simulink model "HESS"  (R2023a)
settings: Solver=daessc  StartTime=0.0  StopTime=2474  MaxStep=0.1  RelTol=1e-3
undefined symbols (not defined in the file or in its folder): Battery, Capacitor, Ri
libraries: fl_lib x31, nesl_utility x18, batteryecm_lib x1, rllib x1
settings Model: Creator=antaeug  LastModifiedBy=antaeug

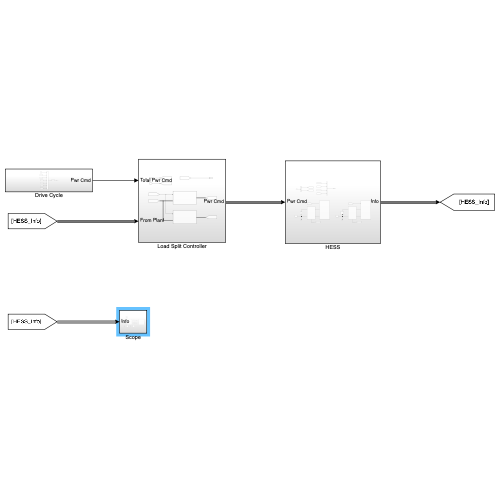
[thumbnail: Simulink's stored preview of the top-level diagram]
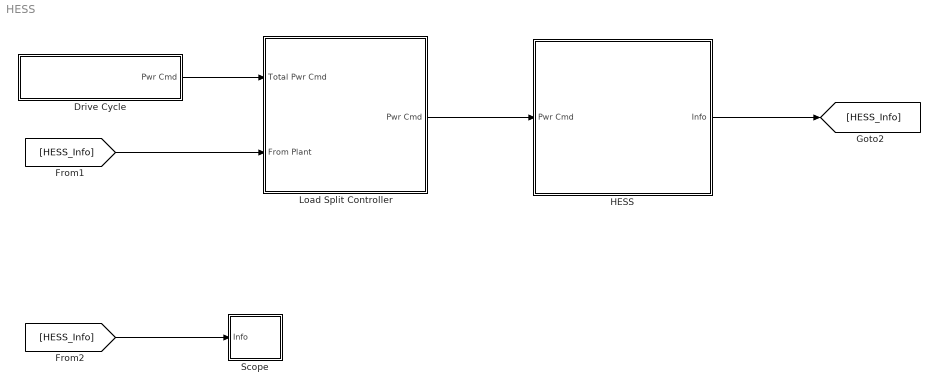
== system HESS ==
  Drive Cycle : Subsystem
  HESS : Subsystem
  Load Split Controller : Subsystem
  Scope : Subsystem
  wires:
  Drive Cycle/1(Pwr Cmd) -> Load Split Controller/1(Total Pwr Cmd)
  Load Split Controller/1(Pwr Cmd) -> HESS/1(Pwr Cmd)
  HESS/1(Info) -> [HESS_Info]
  [HESS_Info] -> Scope/1(Info)
  [HESS_Info] -> Load Split Controller/2(From Plant)

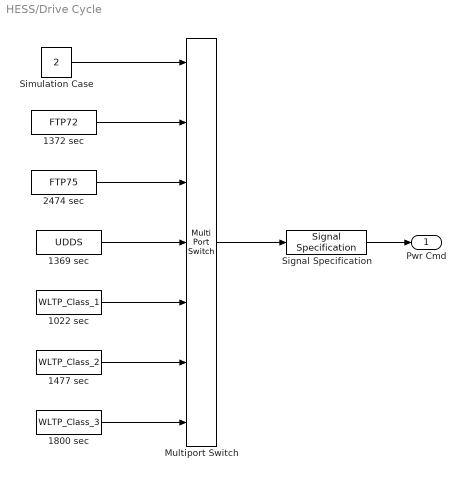
== system HESS/Drive Cycle ==
  1022 sec : FromWorkspace  VariableName=WLTP_Class_1  Interpolate=off  ZeroCross=off  OutputAfterFinalValue=Setting to zero
  1369 sec : FromWorkspace  VariableName=UDDS  Interpolate=off  ZeroCross=off  OutputAfterFinalValue=Setting to zero
  1372 sec : FromWorkspace  VariableName=FTP72  Interpolate=off  ZeroCross=off  OutputAfterFinalValue=Setting to zero
  1477 sec : FromWorkspace  VariableName=WLTP_Class_2  Interpolate=off  ZeroCross=off  OutputAfterFinalValue=Setting to zero
  1800 sec : FromWorkspace  VariableName=WLTP_Class_3  Interpolate=off  ZeroCross=off  OutputAfterFinalValue=Setting to zero
  2474 sec : FromWorkspace  VariableName=FTP75  Interpolate=off  ZeroCross=off  OutputAfterFinalValue=Setting to zero
  Multiport Switch : MultiPortSwitch  Inputs=6  SaturateOnIntegerOverflow=off  InputSameDT=off
  Signal Specification : SignalSpecification  Unit=W
  Simulation Case : Constant  Value=2
  Pwr Cmd : Outport
  wires:
  1372 sec/1 -> Multiport Switch/2
  Signal Specification/1 -> Pwr Cmd/1
  Multiport Switch/1 -> Signal Specification/1
  Simulation Case/1 -> Multiport Switch/1
  2474 sec/1 -> Multiport Switch/3
  1369 sec/1 -> Multiport Switch/4
  1477 sec/1 -> Multiport Switch/6
  1022 sec/1 -> Multiport Switch/5
  1800 sec/1 -> Multiport Switch/7

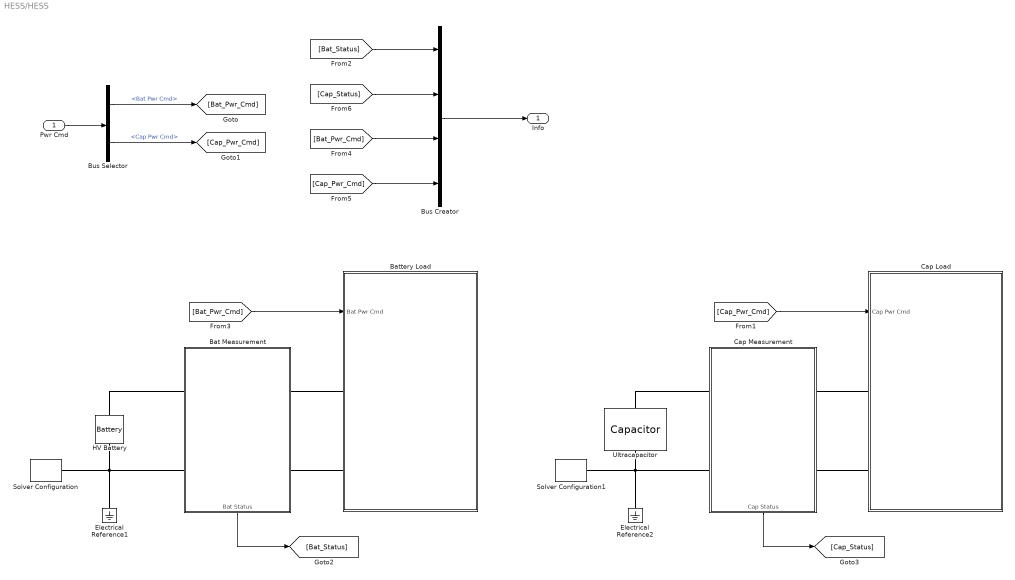
== system HESS/HESS ==
  Pwr Cmd : Inport
  Bat Measurement : Subsystem
      settings: PortSchema="{\"entries\":[{\"content\":{\"sides\":[{\"content\":{\"connectorIds\":[\"LConn1\",\"LConn2\"]},\"type\":\"ConnectorPlacement.EquallySpacedRectSide\",\"uuid\":\"d922d1f1-019d-451f-8be4-16b01e818775\"},{\"content\":{\"connectorIds\":[\"RConn1\",\"RConn2\"],\"side\":\"RIGHT\"},\"type\":\"ConnectorPlacement.EquallySpacedRectSide\",\"uuid\":\"6462d40f-4676-4bff-8e25-5b847feb4e24\"},{\"content\":{\"side\":\"TOP\"},\"type\":\"ConnectorPlacement.EquallySpacedRectSide\",\"uuid\":\"03ad4d94-013a-4b50-b094-3d1359848380\"},{\"content\":{\"connectorIds\":[\"Out1\"],\"side\":\"BOTTOM\"},\"type\":\"ConnectorPlacement.EquallySpacedRectSide\",\"uuid\":\"1e4082bc-bf86-4ee6-a4f5-78f09401198d\"}]},\"type\":\"ConnectorPlacement.EquallySpacedConnector\",\"uuid\":\"2964760f-0df3-43f8-9aa6-d9b794f3ad37\"}],\"packageUris\":[\"http://schema.mathworks.com/mf0/Connector/R2020b\"],\"version\":\"1.0\"}"
  Battery Load : Subsystem
  Bus Creator : BusCreator  Inputs=4
  Bus Selector : BusSelector  OutputSignals=Bat Pwr Cmd,Cap Pwr Cmd
  Cap Load : Subsystem
  Cap Measurement : Subsystem
      settings: PortSchema="{\"entries\":[{\"content\":{\"sides\":[{\"content\":{\"connectorIds\":[\"LConn1\",\"LConn2\"]},\"type\":\"ConnectorPlacement.EquallySpacedRectSide\",\"uuid\":\"d922d1f1-019d-451f-8be4-16b01e818775\"},{\"content\":{\"connectorIds\":[\"RConn1\",\"RConn2\"],\"side\":\"RIGHT\"},\"type\":\"ConnectorPlacement.EquallySpacedRectSide\",\"uuid\":\"6462d40f-4676-4bff-8e25-5b847feb4e24\"},{\"content\":{\"side\":\"TOP\"},\"type\":\"ConnectorPlacement.EquallySpacedRectSide\",\"uuid\":\"03ad4d94-013a-4b50-b094-3d1359848380\"},{\"content\":{\"connectorIds\":[\"Out1\"],\"side\":\"BOTTOM\"},\"type\":\"ConnectorPlacement.EquallySpacedRectSide\",\"uuid\":\"1e4082bc-bf86-4ee6-a4f5-78f09401198d\"}]},\"type\":\"ConnectorPlacement.EquallySpacedConnector\",\"uuid\":\"2964760f-0df3-43f8-9aa6-d9b794f3ad37\"}],\"packageUris\":[\"http://schema.mathworks.com/mf0/Connector/R2020b\"],\"version\":\"1.0\"}"
  Electrical Reference1 : fl_lib/Electrical/Electrical Elements/Electrical Reference
  Electrical Reference2 : fl_lib/Electrical/Electrical Elements/Electrical Reference
  HV Battery : batteryecm_lib/Battery  Vnom=Battery.NominalVoltage V  prm_dir=1  R1_dis=2 Ohm  R1_ch=2 Ohm  R1=Battery.InternalResistance Ohm  prm_AH=2  AH=Battery.Capacity hr*A  V1=Battery.V1 V  AH1=Battery.AH1 hr*A  prm_R2=1  R2=2000 Ohm  Tmeas=25 degC  charge_measurement_port=simscape.enum.battery.enable.no  prm_dyn=1  Rp1=0.005 Ohm  tau1=30 s  Rp2=0.005 Ohm  tau2=30 s  Rp3=0.005 Ohm  tau3=30 s  Rp4=0.005 Ohm  tau4=30 s  Rp5=0.005 Ohm  tau5=30 s  prm_fade=1  N_fade=100  AH_fade=45 hr*A  R1_fade=2.02 Ohm  R1_ch_fade=2.02 Ohm  V1_fade=10.35 V  prm_age=1  prm_age_OCV=1  OCV_age=0.9  SOC_age=60  Tmeas_age=298.15 K  delta_time_age_vec=[0] d  temperature_age_vec=[273] K  OCV_scaling_age=2.2134e6  OCV_offset_age=1.632e6  temp_exp_age=0.515833569 V  t_exp_age=0.75  Vnom_T2=Vnom V  R1_T2=Ri+0.1*Ri Ohm  R1_T2_dis=2.2 Ohm  R1_T2_ch=2.2 Ohm  V1_T2=V1 V  R2_T2=2200 Ohm  Rp1_T2=0.005 Ohm  tau1_T2=30 s  Rp2_T2=0.005 Ohm  tau2_T2=30 s  Rp3_T2=0.005 Ohm  tau3_T2=30 s  Rp4_T2=0.005 Ohm  tau4_T2=30 s  Rp5_T2=0.005 Ohm  tau5_T2=30 s  Tmeas2=0 degC  thermal_port=simscape.enum.thermaleffects.omit  thermal_mass=89400 J/K  i_specify=off  i_priority=None  i=0 A  i_nominal_specify=off  i_nominal_unit=A  i_nominal_value=1  v_specify=off  v_priority=None  v=0 V  v_nominal_specify=off  v_nominal_unit=V  v_nominal_value=1  charge_specify=on  charge_priority=High  charge=Battery.InitialCharge hr*A  charge_nominal_specify=off  charge_nominal_unit=A*hr  charge_nominal_value=1  num_cycles_specify=off  num_cycles_priority=High  num_cycles=0  num_cycles_nominal_specify=off  num_cycles_nominal_unit=1  num_cycles_nominal_value=1  temperature_specify=on  temperature_priority=High  temperature=25 degC  temperature_nominal_specify=off  temperature_nominal_unit=K  temperature_nominal_value=1
  Solver Configuration : nesl_utility/Solver Configuration  PhysicalDomain=network_engine_domain  SubClassName=solver  LeftPortType=input  RightPortType=generic  Tones=[]  Harmonics=[]  SimulateNoise=off  Profile=off  UseLocalSampling=off  EnableSwitchedLinearOptims=on  FrequencyDomain=off  UseCCode=off  RelTol=0.001  AbsTol=1e-06  MinStep=1e-09  ToWorkspace=off  RevertToSquareIcSolve=off  NumHomotopyIterations=100  PhasorMode=off  PhasorModeNumHarmonics=1  ConsistencySolver=NEWTON_FTOL  IndexReductionMethod=DerivativeReplacement  DoDC=off  ResidualTolerance=1e-09  ConsistencyTolSource=GLOBAL  ConsistencyAbsTol=0.001  ConsistencyRelTol=0.001  ConsistencyTolFactor=0.001  UseLocalSolver=on  LocalSolverChoice=NE_BACKWARD_EULER_ADVANCER  ResolveIndetEquations=on  FunctionEvalNumThread=1  LocalSolverSampleTime=0.01  DoFixedCost=on  MaxNonlinIter=3  MaxModeIter=2  ComputeImpulses=off  ImpulseIterations=2  LinearAlgebra=auto  LinearAlgebraNumThread=0  EquationFormulation=NE_TIME_EF  DelaysMemoryBudget=1024  AutomaticFiltering=on  FilteringTimeConstant=0.001  PartitionStorageMethod=AS_NEEDED  PartitionMemoryBudget=1024  PartitionMethod=FAST
  Solver Configuration1 : nesl_utility/Solver Configuration  PhysicalDomain=network_engine_domain  SubClassName=solver  LeftPortType=input  RightPortType=generic  Tones=[]  Harmonics=[]  SimulateNoise=off  Profile=off  UseLocalSampling=off  EnableSwitchedLinearOptims=on  FrequencyDomain=off  UseCCode=off  RelTol=0.001  AbsTol=1e-06  MinStep=1e-09  ToWorkspace=off  RevertToSquareIcSolve=off  NumHomotopyIterations=100  PhasorMode=off  PhasorModeNumHarmonics=1  ConsistencySolver=NEWTON_FTOL  IndexReductionMethod=DerivativeReplacement  DoDC=off  ResidualTolerance=1e-09  ConsistencyTolSource=GLOBAL  ConsistencyAbsTol=0.001  ConsistencyRelTol=0.001  ConsistencyTolFactor=0.001  UseLocalSolver=on  LocalSolverChoice=NE_BACKWARD_EULER_ADVANCER  ResolveIndetEquations=on  FunctionEvalNumThread=1  LocalSolverSampleTime=0.01  DoFixedCost=on  MaxNonlinIter=3  MaxModeIter=2  ComputeImpulses=off  ImpulseIterations=2  LinearAlgebra=auto  LinearAlgebraNumThread=0  EquationFormulation=NE_TIME_EF  DelaysMemoryBudget=1024  AutomaticFiltering=on  FilteringTimeConstant=0.001  PartitionStorageMethod=AS_NEEDED  PartitionMemoryBudget=1024  PartitionMethod=FAST
  Ultracapacitor : fl_lib/Electrical/Electrical Elements/Capacitor  c=Capacitor.Capacitance F  r=Capacitor.InternalResistance mOhm  g=0 1/Ohm  i_specify=off  i_priority=None  i=20 A  i_nominal_specify=off  i_nominal_unit=A  i_nominal_value=1  v_specify=off  v_priority=None  v=600 V  v_nominal_specify=off  v_nominal_unit=V  v_nominal_value=1  vc_specify=on  vc_priority=None  vc=Capacitor.Voltage V  vc_nominal_specify=off  vc_nominal_unit=V  vc_nominal_value=600
  Info : Outport
  wires:
  Pwr Cmd/1 -> Bus Selector/1
  Bus Selector/1 -> [Bat_Pwr_Cmd]  "<Bat Pwr Cmd>"
  Bus Selector/2 -> [Cap_Pwr_Cmd]  "<Cap Pwr Cmd>"
  [Bat_Status] -> Bus Creator/1
  Bus Creator/1 -> Info/1
  [Cap_Pwr_Cmd] -> Bus Creator/4
  [Bat_Pwr_Cmd] -> Bus Creator/3
  Bat Measurement/1(Bat Status) -> [Bat_Status]
  [Bat_Pwr_Cmd] -> Battery Load/1(Bat Pwr Cmd)
  Cap Measurement/1(Cap Status) -> [Cap_Status]
  [Cap_Pwr_Cmd] -> Cap Load/1(Cap Pwr Cmd)
  [Cap_Status] -> Bus Creator/2
  connections:
  HV Battery/RConn1 -- Bat Measurement/LConn2 -- Solver Configuration/RConn1 -- Electrical Reference1/LConn1
  Bat Measurement/LConn1 -- HV Battery/LConn1
  Battery Load/LConn1 -- Bat Measurement/RConn1
  Battery Load/LConn2 -- Bat Measurement/RConn2
  Electrical Reference2/LConn1 -- Ultracapacitor/RConn1 -- Cap Measurement/LConn2 -- Solver Configuration1/RConn1
  Ultracapacitor/LConn1 -- Cap Measurement/LConn1
  Cap Load/LConn2 -- Cap Measurement/RConn2
  Cap Load/LConn1 -- Cap Measurement/RConn1

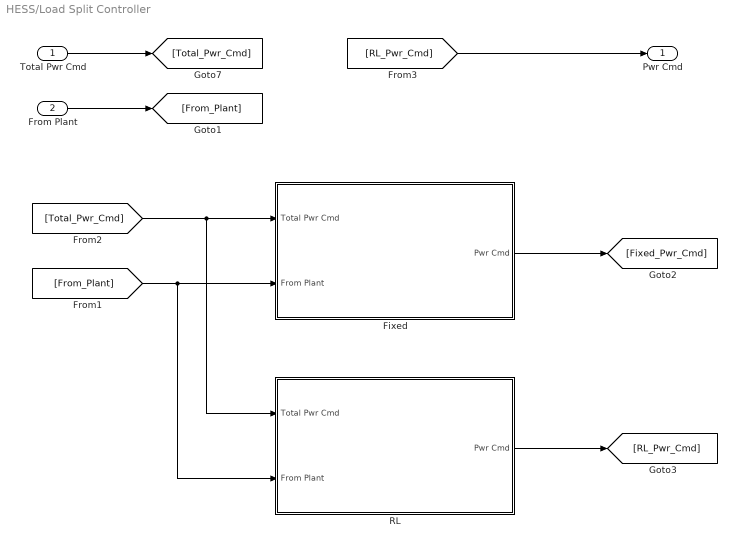
== system HESS/Load Split Controller ==
  Total Pwr Cmd : Inport
  From Plant : Inport  Port=2
  Fixed : Subsystem
  RL : Subsystem
  Pwr Cmd : Outport
  wires:
  [Total_Pwr_Cmd] -> RL/1(Total Pwr Cmd), Fixed/1(Total Pwr Cmd)
  [From_Plant] -> RL/2(From Plant), Fixed/2(From Plant)
  Fixed/1(Pwr Cmd) -> [Fixed_Pwr_Cmd]
  RL/1(Pwr Cmd) -> [RL_Pwr_Cmd]
  Total Pwr Cmd/1 -> [Total_Pwr_Cmd]
  From Plant/1 -> [From_Plant]
  [RL_Pwr_Cmd] -> Pwr Cmd/1

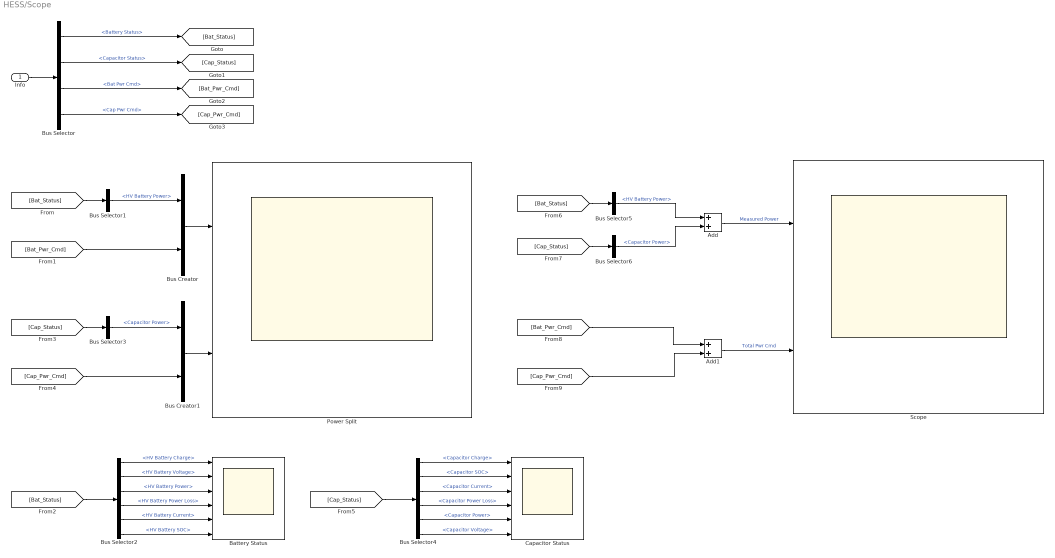
== system HESS/Scope ==
  Info : Inport
  Add : Sum
  Add1 : Sum
  Battery Status : Scope  NumInputPorts=6
  Bus Creator : BusCreator  Inputs=2
  Bus Creator1 : BusCreator  Inputs=2
  Bus Selector : BusSelector  OutputSignals=Battery Status,Capacitor Status,Bat Pwr Cmd,Cap Pwr Cmd
  Bus Selector1 : BusSelector  OutputSignals=HV Battery Power
  Bus Selector2 : BusSelector  OutputSignals=HV Battery Charge,HV Battery Voltage,HV Battery Power,HV Battery Power Loss,HV Battery Current,HV Battery SOC
  Bus Selector3 : BusSelector  OutputSignals=Capacitor Power
  Bus Selector4 : BusSelector  OutputSignals=Capacitor Charge,Capacitor SOC,Capacitor Current,Capacitor Power Loss,Capacitor Power,Capacitor Voltage
  Bus Selector5 : BusSelector  OutputSignals=HV Battery Power
  Bus Selector6 : BusSelector  OutputSignals=Capacitor Power
  Capacitor Status : Scope  NumInputPorts=6
  Power Split : Scope  NumInputPorts=2
  Scope : Scope  NumInputPorts=2
  wires:
  Info/1 -> Bus Selector/1
  Bus Selector/1 -> [Bat_Status]  "<Battery Status>"
  [Bat_Status] -> Bus Selector1/1
  Bus Selector1/1 -> Bus Creator/1  "<HV Battery Power>"
  [Bat_Pwr_Cmd] -> Bus Creator/2
  Bus Selector/3 -> [Bat_Pwr_Cmd]  "<Bat Pwr Cmd>"
  Bus Selector/4 -> [Cap_Pwr_Cmd]  "<Cap Pwr Cmd>"
  [Bat_Status] -> Bus Selector2/1
  Bus Selector2/1 -> Battery Status/1  "<HV Battery Charge>"
  Bus Selector2/2 -> Battery Status/2  "<HV Battery Voltage>"
  Bus Selector2/3 -> Battery Status/3  "<HV Battery Power>"
  Bus Selector2/4 -> Battery Status/4  "<HV Battery Power Loss>"
  Bus Selector2/5 -> Battery Status/5  "<HV Battery Current>"
  Bus Selector2/6 -> Battery Status/6  "<HV Battery SOC>"
  Bus Selector3/1 -> Bus Creator1/1  "<Capacitor Power>"
  [Cap_Status] -> Bus Selector3/1
  [Cap_Pwr_Cmd] -> Bus Creator1/2
  Bus Selector/2 -> [Cap_Status]  "<Capacitor Status>"
  Bus Creator/1 -> Power Split/1
  Bus Creator1/1 -> Power Split/2
  Bus Selector4/6 -> Capacitor Status/6  "<Capacitor Voltage>"
  Bus Selector4/1 -> Capacitor Status/1  "<Capacitor Charge>"
  Bus Selector4/2 -> Capacitor Status/2  "<Capacitor SOC>"
  Bus Selector4/3 -> Capacitor Status/3  "<Capacitor Current>"
  Bus Selector4/4 -> Capacitor Status/4  "<Capacitor Power Loss>"
  Bus Selector4/5 -> Capacitor Status/5  "<Capacitor Power>"
  [Cap_Status] -> Bus Selector4/1
  Bus Selector5/1 -> Add/1  "<HV Battery Power>"
  [Bat_Status] -> Bus Selector5/1
  Bus Selector6/1 -> Add/2  "<Capacitor Power>"
  [Cap_Status] -> Bus Selector6/1
  [Bat_Pwr_Cmd] -> Add1/1
  [Cap_Pwr_Cmd] -> Add1/2
  Add/1 -> Scope/1  "Measured Power"
  Add1/1 -> Scope/2  "Total Pwr Cmd"

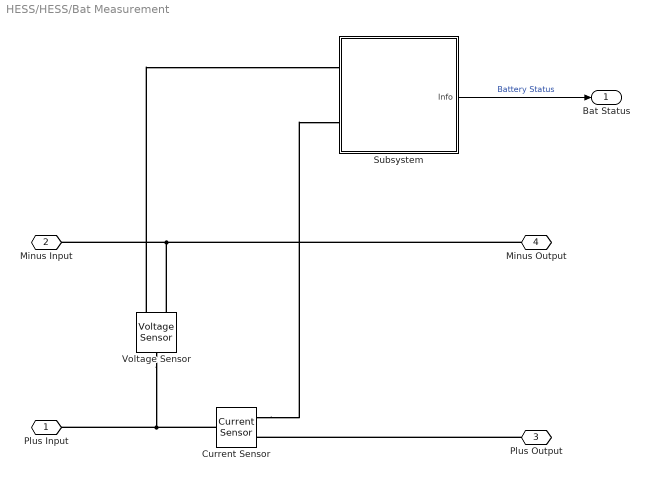
== system HESS/HESS/Bat Measurement ==
  Current Sensor : fl_lib/Electrical/Electrical Sensors/Current Sensor
  Subsystem : Subsystem
  Voltage Sensor : fl_lib/Electrical/Electrical Sensors/Voltage Sensor
  Plus Input : PMIOPort  Side=Left
  Minus Input : PMIOPort  Port=2  Side=Left
  Plus Output : PMIOPort  Port=3  Side=Right
  Minus Output : PMIOPort  Port=4  Side=Right
  Bat Status : Outport
  wires:
  Subsystem/1(Info) -> Bat Status/1  "Battery Status"
  connections:
  Voltage Sensor/RConn2 -- Minus Input/RConn1 -- Minus Output/RConn1
  Current Sensor/LConn1 -- Voltage Sensor/LConn1 -- Plus Input/RConn1
  Voltage Sensor/RConn1 -- Subsystem/LConn1
  Current Sensor/RConn1 -- Subsystem/LConn2
  Plus Output/RConn1 -- Current Sensor/RConn2

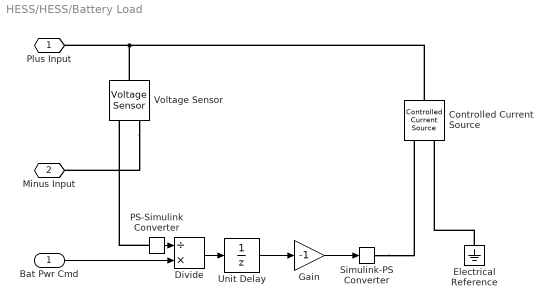
== system HESS/HESS/Battery Load ==
  Bat Pwr Cmd : Inport
  Controlled Current Source : fl_lib/Electrical/Electrical Sources/Controlled Current Source
  Divide : Product  Inputs=/*
  Electrical Reference : fl_lib/Electrical/Electrical Elements/Electrical Reference
  Gain : Gain  Gain=-1
  PS-Simulink Converter : nesl_utility/PS-Simulink Converter  PhysicalDomain=network_engine_domain  SubClassName=ps_output  LeftPortType=input  RightPortType=output  PseudoPeriodic=off  Frequencies=[]  VectorFormat=inherit  Unit=V  AffineConversion=off
  Simulink-PS Converter : nesl_utility/Simulink-PS Converter  PhysicalDomain=network_engine_domain  SubClassName=ps_input  LeftPortType=input  RightPortType=output  PseudoPeriodic=off  Frequencies=[]  NoiseDistribution=none  NoiseParameters=[]  Unit=A  AffineConversion=off  FilteringAndDerivatives=provide  SimscapeFilterOrder=1  InputFilterTimeConstant=0.001  UdotUserProvided=0
  Unit Delay : UnitDelay  SampleTime=-1  HasFrameUpgradeWarning=on
  Voltage Sensor : fl_lib/Electrical/Electrical Sensors/Voltage Sensor
  Plus Input : PMIOPort  Side=Left
  Minus Input : PMIOPort  Port=2  Side=Left
  wires:
  PS-Simulink Converter/1 -> Divide/1
  Bat Pwr Cmd/1 -> Divide/2
  Divide/1 -> Unit Delay/1
  Unit Delay/1 -> Gain/1
  Gain/1 -> Simulink-PS Converter/1
  connections:
  Electrical Reference/LConn1 -- Controlled Current Source/RConn2
  Controlled Current Source/LConn1 -- Voltage Sensor/LConn1 -- Plus Input/RConn1
  Voltage Sensor/RConn2 -- Minus Input/RConn1
  PS-Simulink Converter/LConn1 -- Voltage Sensor/RConn1
  Simulink-PS Converter/RConn1 -- Controlled Current Source/RConn1

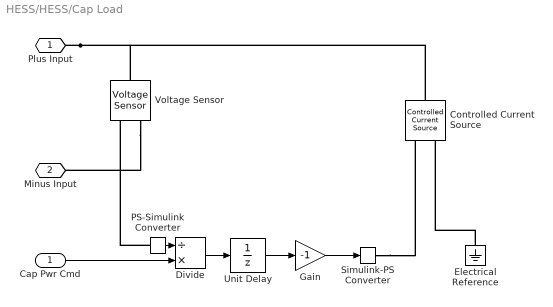
== system HESS/HESS/Cap Load ==
  Cap Pwr Cmd : Inport
  Controlled Current Source : fl_lib/Electrical/Electrical Sources/Controlled Current Source
  Divide : Product  Inputs=/*
  Electrical Reference : fl_lib/Electrical/Electrical Elements/Electrical Reference
  Gain : Gain  Gain=-1
  PS-Simulink Converter : nesl_utility/PS-Simulink Converter  PhysicalDomain=network_engine_domain  SubClassName=ps_output  LeftPortType=input  RightPortType=output  PseudoPeriodic=off  Frequencies=[]  VectorFormat=inherit  Unit=V  AffineConversion=off
  Simulink-PS Converter : nesl_utility/Simulink-PS Converter  PhysicalDomain=network_engine_domain  SubClassName=ps_input  LeftPortType=input  RightPortType=output  PseudoPeriodic=off  Frequencies=[]  NoiseDistribution=none  NoiseParameters=[]  Unit=A  AffineConversion=off  FilteringAndDerivatives=provide  SimscapeFilterOrder=1  InputFilterTimeConstant=0.001  UdotUserProvided=0
  Unit Delay : UnitDelay  SampleTime=-1  HasFrameUpgradeWarning=on
  Voltage Sensor : fl_lib/Electrical/Electrical Sensors/Voltage Sensor
  Plus Input : PMIOPort  Side=Left
  Minus Input : PMIOPort  Port=2  Side=Left
  wires:
  PS-Simulink Converter/1 -> Divide/1
  Cap Pwr Cmd/1 -> Divide/2
  Divide/1 -> Unit Delay/1
  Unit Delay/1 -> Gain/1
  Gain/1 -> Simulink-PS Converter/1
  connections:
  Electrical Reference/LConn1 -- Controlled Current Source/RConn2
  Plus Input/RConn1 -- Controlled Current Source/LConn1 -- Voltage Sensor/LConn1
  Voltage Sensor/RConn2 -- Minus Input/RConn1
  PS-Simulink Converter/LConn1 -- Voltage Sensor/RConn1
  Simulink-PS Converter/RConn1 -- Controlled Current Source/RConn1

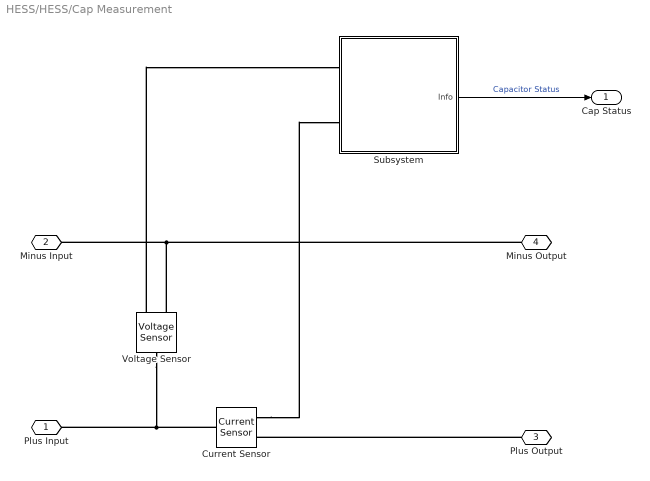
== system HESS/HESS/Cap Measurement ==
  Current Sensor : fl_lib/Electrical/Electrical Sensors/Current Sensor
  Subsystem : Subsystem
  Voltage Sensor : fl_lib/Electrical/Electrical Sensors/Voltage Sensor
  Plus Input : PMIOPort  Side=Left
  Minus Input : PMIOPort  Port=2  Side=Left
  Plus Output : PMIOPort  Port=3  Side=Right
  Minus Output : PMIOPort  Port=4  Side=Right
  Cap Status : Outport
  wires:
  Subsystem/1(Info) -> Cap Status/1  "Capacitor Status"
  connections:
  Minus Output/RConn1 -- Voltage Sensor/RConn2 -- Minus Input/RConn1
  Current Sensor/LConn1 -- Voltage Sensor/LConn1 -- Plus Input/RConn1
  Voltage Sensor/RConn1 -- Subsystem/LConn1
  Current Sensor/RConn1 -- Subsystem/LConn2
  Plus Output/RConn1 -- Current Sensor/RConn2

== system HESS/Load Split Controller/Fixed ==
  Total Pwr Cmd : Inport
  From Plant : Inport  Port=2
  Add : Sum  Inputs=+-
  Bus Creator : BusCreator  Inputs=2
  Gain : Gain  Gain=0.9
  Terminator : Terminator
  Pwr Cmd : Outport
  wires:
  Gain/1 -> Add/2, Bus Creator/1  "Bat Pwr Cmd"
  Add/1 -> Bus Creator/2  "Cap Pwr Cmd"
  Bus Creator/1 -> Pwr Cmd/1
  Total Pwr Cmd/1 -> Add/1, Gain/1
  From Plant/1 -> Terminator/1

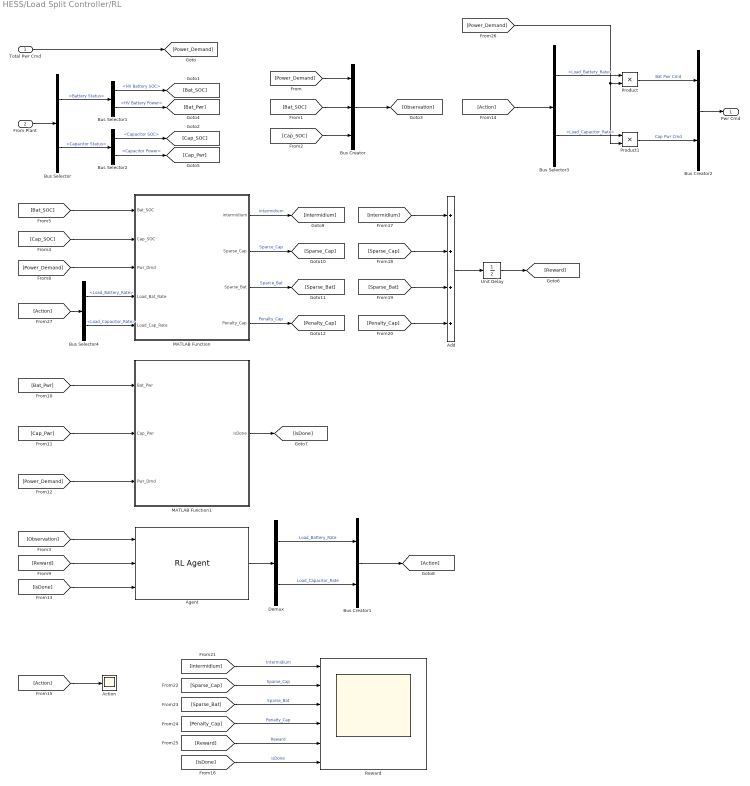
== system HESS/Load Split Controller/RL ==
  Total Pwr Cmd : Inport
  From Plant : Inport  Port=2
  Action : Scope
  Add : Sum  Inputs=++++
  Agent : rllib/RL Agent  Agent=agent  ExternalActionAsInput=off  ProvideLastAction=off  ProvideCumRwd=off  TreatAsDirectFeedthrough=on  UseStrictObservationDataTypes=off
  Bus Creator : BusCreator  Inputs=3
  Bus Creator1 : BusCreator  Inputs=2
  Bus Creator2 : BusCreator  Inputs=2
  Bus Selector : BusSelector  OutputSignals=Battery Status,Capacitor Status
  Bus Selector1 : BusSelector  OutputSignals=HV Battery SOC,HV Battery Power
  Bus Selector2 : BusSelector  OutputSignals=Capacitor SOC,Capacitor Power
  Bus Selector3 : BusSelector  OutputSignals=Load_Battery_Rate,Load_Capacitor_Rate
  Bus Selector4 : BusSelector  OutputSignals=Load_Battery_Rate,Load_Capacitor_Rate
  Demux : Demux  Outputs=2
  MATLAB Function : MATLAB Function  TreatAsAtomicUnit=on
  MATLAB Function1 : MATLAB Function  TreatAsAtomicUnit=on
  Product : Product
  Product1 : Product
  Reward : Scope  NumInputPorts=6
  Unit Delay : UnitDelay  SampleTime=-1  HasFrameUpgradeWarning=on
  Pwr Cmd : Outport
  wires:
  Agent/1 -> Demux/1
  From Plant/1 -> Bus Selector/1
  Total Pwr Cmd/1 -> [Power_Demand]
  Bus Selector/1 -> Bus Selector1/1  "<Battery Status>"
  Bus Selector/2 -> Bus Selector2/1  "<Capacitor Status>"
  Bus Selector1/1 -> [Bat_SOC]  "<HV Battery SOC>"
  [Power_Demand] -> Bus Creator/1
  [Bat_SOC] -> Bus Creator/2
  [Cap_SOC] -> Bus Creator/3
  Bus Creator/1 -> [Observation]
  [Observation] -> Agent/1
  Demux/1 -> Bus Creator1/1  "Load_Battery_Rate"
  Demux/2 -> Bus Creator1/2  "Load_Capacitor_Rate"
  Bus Selector1/2 -> [Bat_Pwr]  "<HV Battery Power>"
  Bus Selector2/1 -> [Cap_SOC]  "<Capacitor SOC>"
  Bus Selector2/2 -> [Cap_Pwr]  "<Capacitor Power>"
  Bus Creator1/1 -> [Action]
  [Cap_SOC] -> MATLAB Function/2(Cap_SOC)
  [Bat_SOC] -> MATLAB Function/1(Bat_SOC)
  [Power_Demand] -> MATLAB Function/3(Pwr_Dmd)
  MATLAB Function/1(intermidium) -> [Intermidium]  "intermidium"
  [Reward] -> Agent/2
  [Bat_Pwr] -> MATLAB Function1/1(Bat_Pwr)
  [Cap_Pwr] -> MATLAB Function1/2(Cap_Pwr)
  [Power_Demand] -> MATLAB Function1/3(Pwr_Dmd)
  MATLAB Function1/1(isDone) -> [isDone]
  [isDone] -> Agent/3
  [Action] -> Bus Selector3/1
  [Action] -> Action/1
  MATLAB Function/2(Sparse_Cap) -> [Sparse_Cap]  "Sparce_Cap"
  MATLAB Function/3(Sparse_Bat) -> [Sparse_Bat]  "Sparce_Bat"
  MATLAB Function/4(Penalty_Cap) -> [Penalty_Cap]  "Penalty_Cap"
  [Intermidium] -> Add/1
  [Sparse_Cap] -> Add/2
  [Sparse_Bat] -> Add/3
  [Penalty_Cap] -> Add/4
  [Intermidium] -> Reward/1  "Intermidium"
  [Sparse_Cap] -> Reward/2  "Sparse_Cap"
  [Sparse_Bat] -> Reward/3  "Sparse_Bat"
  [Penalty_Cap] -> Reward/4  "Penalty_Cap"
  [Reward] -> Reward/5  "Reward"
  Bus Selector3/1 -> Product/1  "<Load_Battery_Rate>"
  [Power_Demand] -> Product1/2, Product/2
  Bus Selector3/2 -> Product1/1  "<Load_Capacitor_Rate>"
  Product/1 -> Bus Creator2/1  "Bat Pwr Cmd"
  Product1/1 -> Bus Creator2/2  "Cap Pwr Cmd"
  Bus Creator2/1 -> Pwr Cmd/1
  [isDone] -> Reward/6  "isDone"
  Bus Selector4/1 -> MATLAB Function/4(Load_Bat_Rate)  "<Load_Battery_Rate>"
  Bus Selector4/2 -> MATLAB Function/5(Load_Cap_Rate)  "<Load_Capacitor_Rate>"
  [Action] -> Bus Selector4/1
  Add/1 -> Unit Delay/1
  Unit Delay/1 -> [Reward]

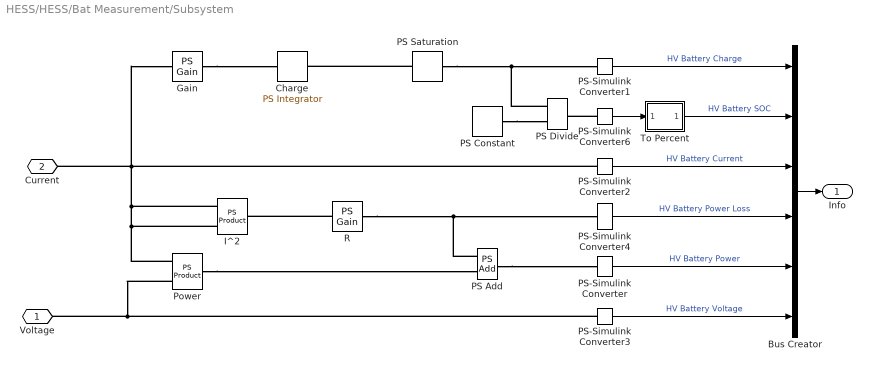
== system HESS/HESS/Bat Measurement/Subsystem ==
  Bus Creator : BusCreator  Inputs=6
  Charge : fl_lib/Physical Signals/Linear Operators/PS Integrator  reset_method=foundation.enum.IntegratorResetSpec.None  initial_condition_spec=foundation.enum.IntegratorICSpec.Internal  saturation_spec=foundation.enum.IntegratorSaturationSpec.None  saturation_source_spec=foundation.enum.IntegratorSaturationSourceSpec.Internal  x0=Battery.InitialCharge A*hr  xu=inf s  xl=-inf s
      settings: AttributesFormatString=%<x0> [%<x0_unit>]
  Gain : fl_lib/Physical Signals/Functions/PS Gain  gain=-1
      settings: AttributesFormatString=%<gain>
  I^2 : fl_lib/Physical Signals/Functions/PS Product
  PS Add : fl_lib/Physical Signals/Functions/PS Add
  PS Constant : fl_lib/Physical Signals/Sources/PS Constant  constant=Battery.Capacity A*hr
      settings: AttributesFormatString=%<constant> [%<constant_unit>]
  PS Divide : fl_lib/Physical Signals/Functions/PS Divide
  PS Saturation : fl_lib/Physical Signals/Nonlinear Operators/PS Saturation  upper_limit=Battery.Capacity A*hr  lower_limit=0 A*hr
      settings: AttributesFormatString=|
      | Upper: %<upper_limit>
      | Lower: %<lower_limit>
  PS-Simulink Converter : nesl_utility/PS-Simulink Converter  PhysicalDomain=network_engine_domain  SubClassName=ps_output  LeftPortType=input  RightPortType=output  PseudoPeriodic=off  Frequencies=[]  VectorFormat=1-D array  Unit=W  AffineConversion=off
  PS-Simulink Converter1 : nesl_utility/PS-Simulink Converter  PhysicalDomain=network_engine_domain  SubClassName=ps_output  LeftPortType=input  RightPortType=output  PseudoPeriodic=off  Frequencies=[]  VectorFormat=1-D array  Unit=A*hr  AffineConversion=off
  PS-Simulink Converter2 : nesl_utility/PS-Simulink Converter  PhysicalDomain=network_engine_domain  SubClassName=ps_output  LeftPortType=input  RightPortType=output  PseudoPeriodic=off  Frequencies=[]  VectorFormat=1-D array  Unit=A  AffineConversion=off
  PS-Simulink Converter3 : nesl_utility/PS-Simulink Converter  PhysicalDomain=network_engine_domain  SubClassName=ps_output  LeftPortType=input  RightPortType=output  PseudoPeriodic=off  Frequencies=[]  VectorFormat=1-D array  Unit=V  AffineConversion=off
  PS-Simulink Converter4 : nesl_utility/PS-Simulink Converter  PhysicalDomain=network_engine_domain  SubClassName=ps_output  LeftPortType=input  RightPortType=output  PseudoPeriodic=off  Frequencies=[]  VectorFormat=1-D array  Unit=W  AffineConversion=off
  PS-Simulink Converter6 : nesl_utility/PS-Simulink Converter  PhysicalDomain=network_engine_domain  SubClassName=ps_output  LeftPortType=input  RightPortType=output  PseudoPeriodic=off  Frequencies=[]  VectorFormat=1-D array  Unit=1  AffineConversion=off
  Power : fl_lib/Physical Signals/Functions/PS Product
  R : fl_lib/Physical Signals/Functions/PS Gain  gain=Battery.InternalResistance Ohm
      settings: AttributesFormatString=%<gain> [%<gain_unit>]
  To Percent : Subsystem
  Voltage : PMIOPort  Side=Left
  Current : PMIOPort  Port=2  Side=Left
  Info : Outport
  wires:
  PS-Simulink Converter4/1 -> Bus Creator/4  "HV Battery Power Loss"
  PS-Simulink Converter3/1 -> Bus Creator/6  "HV Battery Voltage"
  PS-Simulink Converter1/1 -> Bus Creator/1  "HV Battery Charge"
  Bus Creator/1 -> Info/1
  To Percent/1(Out1) -> Bus Creator/2  "HV Battery SOC"
  PS-Simulink Converter/1 -> Bus Creator/5  "HV Battery Power"
  PS-Simulink Converter6/1 -> To Percent/1(In1)
  PS-Simulink Converter2/1 -> Bus Creator/3  "HV Battery Current"
  connections:
  PS Divide/LConn1 -- PS Saturation/RConn1 -- PS-Simulink Converter1/LConn1
  Power/LConn1 -- Voltage/RConn1 -- PS-Simulink Converter3/LConn1
  R/RConn1 -- PS Add/LConn1 -- PS-Simulink Converter4/LConn1
  Power/LConn2 -- I^2/LConn1 -- Current/RConn1 -- Gain/LConn1 -- PS-Simulink Converter2/LConn1 -- I^2/LConn2
  PS Add/RConn1 -- PS-Simulink Converter/LConn1
  R/LConn1 -- I^2/RConn1
  PS Saturation/LConn1 -- Charge/RConn1
  Gain/RConn1 -- Charge/LConn1
  PS-Simulink Converter6/LConn1 -- PS Divide/RConn1
  Power/RConn1 -- PS Add/LConn2
  PS Constant/RConn1 -- PS Divide/LConn2

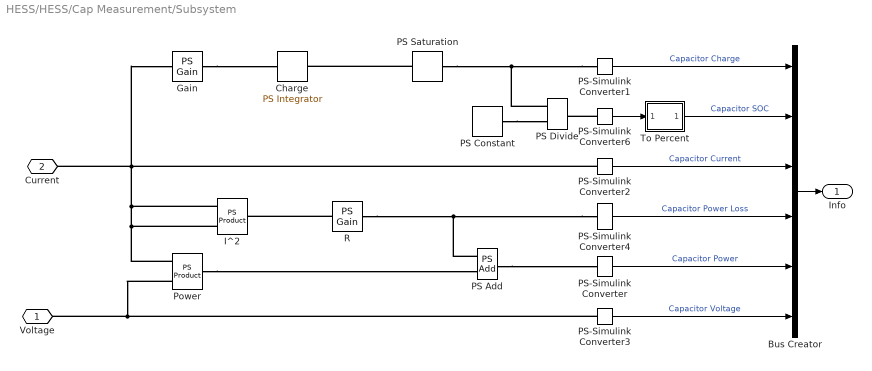
== system HESS/HESS/Cap Measurement/Subsystem ==
  Bus Creator : BusCreator  Inputs=6
  Charge : fl_lib/Physical Signals/Linear Operators/PS Integrator  reset_method=foundation.enum.IntegratorResetSpec.None  initial_condition_spec=foundation.enum.IntegratorICSpec.Internal  saturation_spec=foundation.enum.IntegratorSaturationSpec.None  saturation_source_spec=foundation.enum.IntegratorSaturationSourceSpec.Internal  x0=Capacitor.Capacity A*hr  xu=inf s  xl=-inf s
      settings: AttributesFormatString=%<x0> [%<x0_unit>]
  Gain : fl_lib/Physical Signals/Functions/PS Gain  gain=-1
      settings: AttributesFormatString=%<gain>
  I^2 : fl_lib/Physical Signals/Functions/PS Product
  PS Add : fl_lib/Physical Signals/Functions/PS Add
  PS Constant : fl_lib/Physical Signals/Sources/PS Constant  constant=Capacitor.Capacity A*hr
      settings: AttributesFormatString=%<constant> [%<constant_unit>]
  PS Divide : fl_lib/Physical Signals/Functions/PS Divide
  PS Saturation : fl_lib/Physical Signals/Nonlinear Operators/PS Saturation  upper_limit=Capacitor.Capacity A*hr  lower_limit=0 A*hr
      settings: AttributesFormatString=|
      | Upper: %<upper_limit>
      | Lower: %<lower_limit>
  PS-Simulink Converter : nesl_utility/PS-Simulink Converter  PhysicalDomain=network_engine_domain  SubClassName=ps_output  LeftPortType=input  RightPortType=output  PseudoPeriodic=off  Frequencies=[]  VectorFormat=1-D array  Unit=W  AffineConversion=off
  PS-Simulink Converter1 : nesl_utility/PS-Simulink Converter  PhysicalDomain=network_engine_domain  SubClassName=ps_output  LeftPortType=input  RightPortType=output  PseudoPeriodic=off  Frequencies=[]  VectorFormat=1-D array  Unit=A*hr  AffineConversion=off
  PS-Simulink Converter2 : nesl_utility/PS-Simulink Converter  PhysicalDomain=network_engine_domain  SubClassName=ps_output  LeftPortType=input  RightPortType=output  PseudoPeriodic=off  Frequencies=[]  VectorFormat=1-D array  Unit=A  AffineConversion=off
  PS-Simulink Converter3 : nesl_utility/PS-Simulink Converter  PhysicalDomain=network_engine_domain  SubClassName=ps_output  LeftPortType=input  RightPortType=output  PseudoPeriodic=off  Frequencies=[]  VectorFormat=1-D array  Unit=V  AffineConversion=off
  PS-Simulink Converter4 : nesl_utility/PS-Simulink Converter  PhysicalDomain=network_engine_domain  SubClassName=ps_output  LeftPortType=input  RightPortType=output  PseudoPeriodic=off  Frequencies=[]  VectorFormat=1-D array  Unit=W  AffineConversion=off
  PS-Simulink Converter6 : nesl_utility/PS-Simulink Converter  PhysicalDomain=network_engine_domain  SubClassName=ps_output  LeftPortType=input  RightPortType=output  PseudoPeriodic=off  Frequencies=[]  VectorFormat=1-D array  Unit=1  AffineConversion=off
  Power : fl_lib/Physical Signals/Functions/PS Product
  R : fl_lib/Physical Signals/Functions/PS Gain  gain=Capacitor.InternalResistance Ohm
      settings: AttributesFormatString=%<gain> [%<gain_unit>]
  To Percent : Subsystem
  Voltage : PMIOPort  Side=Left
  Current : PMIOPort  Port=2  Side=Left
  Info : Outport
  wires:
  PS-Simulink Converter4/1 -> Bus Creator/4  "Capacitor Power Loss"
  PS-Simulink Converter3/1 -> Bus Creator/6  "Capacitor Voltage"
  PS-Simulink Converter1/1 -> Bus Creator/1  "Capacitor Charge"
  Bus Creator/1 -> Info/1
  To Percent/1(Out1) -> Bus Creator/2  "Capacitor SOC"
  PS-Simulink Converter/1 -> Bus Creator/5  "Capacitor Power"
  PS-Simulink Converter6/1 -> To Percent/1(In1)
  PS-Simulink Converter2/1 -> Bus Creator/3  "Capacitor Current"
  connections:
  PS-Simulink Converter1/LConn1 -- PS Divide/LConn1 -- PS Saturation/RConn1
  PS-Simulink Converter3/LConn1 -- Power/LConn1 -- Voltage/RConn1
  PS-Simulink Converter4/LConn1 -- R/RConn1 -- PS Add/LConn1
  Current/RConn1 -- Gain/LConn1 -- PS-Simulink Converter2/LConn1 -- I^2/LConn2 -- I^2/LConn1 -- Power/LConn2
  PS Add/RConn1 -- PS-Simulink Converter/LConn1
  R/LConn1 -- I^2/RConn1
  PS Saturation/LConn1 -- Charge/RConn1
  Gain/RConn1 -- Charge/LConn1
  PS-Simulink Converter6/LConn1 -- PS Divide/RConn1
  Power/RConn1 -- PS Add/LConn2
  PS Constant/RConn1 -- PS Divide/LConn2

== system HESS/HESS/Bat Measurement/Subsystem/To Percent ==
  In1 : Inport
  Unit Conversion : UnitConversion
  Out1 : Outport  Unit=%
      settings: AttributesFormatString=%<Unit>
  wires:
  Unit Conversion/1 -> Out1/1
  In1/1 -> Unit Conversion/1

== system HESS/HESS/Cap Measurement/Subsystem/To Percent ==
  In1 : Inport
  Unit Conversion : UnitConversion
  Out1 : Outport  Unit=%
      settings: AttributesFormatString=%<Unit>
  wires:
  Unit Conversion/1 -> Out1/1
  In1/1 -> Unit Conversion/1

== matlab function HESS/Load Split Controller/RL/MATLAB Function1 ==
  data: isDone output; Bat_Pwr input; Cap_Pwr input; Pwr_Dmd input
function isDone = check(Bat_Pwr, Cap_Pwr, Pwr_Dmd)


flag = 0;

if abs(Bat_Pwr + Cap_Pwr - Pwr_Dmd) > 10000
    flag = 1;
end

isDone = flag;

== matlab function HESS/Load Split Controller/RL/MATLAB Function ==
  data: Bat_SOC input; intermidium output; Cap_SOC input; Pwr_Dmd input; Sparse_Cap output; Sparse_Bat output; Penalty_Cap output; Load_Bat_Rate input; Load_Cap_Rate input
function [intermidium, Sparse_Cap, Sparse_Bat, Penalty_Cap] = cal_reward(Bat_SOC, Cap_SOC, Pwr_Dmd, Load_Bat_Rate, Load_Cap_Rate)

Sparse_Cap = 0;
Sparse_Bat = 0;
Penalty_Cap = 0;

Bat_Pwr = Pwr_Dmd * Load_Bat_Rate;
Cap_Pwr = Pwr_Dmd * Load_Cap_Rate;


% Mid reward
intermidium = power(Bat_SOC, 2) + power(Cap_SOC, 2);

% Sparse reward
if (Cap_SOC > 0.65 && Pwr_Dmd > 10000) || (Cap_SOC < 0.65 && Pwr_Dmd < 0)
    tmp = (Pwr_Dmd - Cap_Pwr) / Pwr_Dmd;
    Sparse_Cap = 1 - tmp^0.4;
end

if (Cap_SOC < 0.65 && Pwr_Dmd ~= 0)
    tmp = (Pwr_Dmd - Bat_Pwr) / Pwr_Dmd;
    Sparse_Bat = 1 - tmp^0.4;
end

if (Cap_SOC < 0.65 && Pwr_Dmd > 0)
    tmp = (Pwr_Dmd - Cap_Pwr) / Pwr_Dmd;
    Penalty_Cap = -(1 - tmp^0.4);
end
